simulink model "LAB5T2"  (R2018b)
settings: Solver=VariableStepAuto  StartTime=0.0  StopTime=100  RelTol=1e-3
settings Model: Creator=aloisia  LastModifiedBy=aloisia

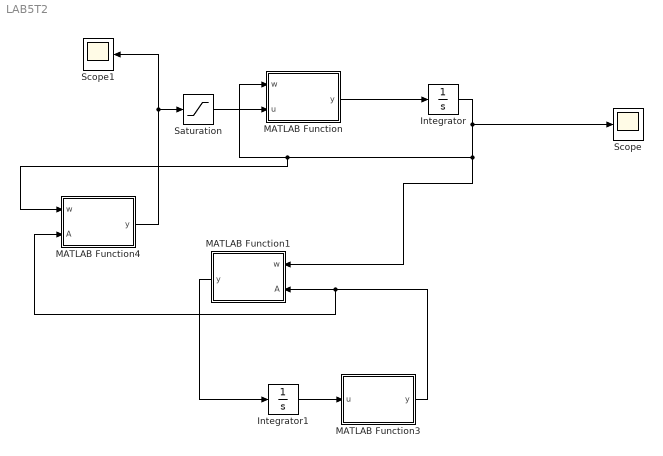
== system LAB5T2 ==
  Integrator : Integrator  InitialCondition=[0; 0; 0.01]
  Integrator1 : Integrator  InitialCondition=[-0.782 0 -0.6233;-0.6233 0 -0.782;0 -1 0]
  MATLAB Function : MATLAB Function  TreatAsAtomicUnit=on
  MATLAB Function1 : MATLAB Function  TreatAsAtomicUnit=on
  MATLAB Function3 : MATLAB Function  TreatAsAtomicUnit=on
  MATLAB Function4 : MATLAB Function  TreatAsAtomicUnit=on
  Saturation : Saturate  UpperLimit=0.01  LowerLimit=0.01
  Scope : Scope
  Scope1 : Scope
  wires:
  MATLAB Function3/1(y) -> MATLAB Function4/2(A), MATLAB Function1/2(A)
  MATLAB Function/1(y) -> Integrator/1
  Integrator1/1 -> MATLAB Function3/1(u)
  Integrator/1 -> MATLAB Function4/1(w), MATLAB Function/1(w), MATLAB Function1/1(w), Scope/1
  MATLAB Function1/1(y) -> Integrator1/1
  MATLAB Function4/1(y) -> Scope1/1, Saturation/1
  Saturation/1 -> MATLAB Function/2(u)

== matlab function LAB5T2/MATLAB Function1 ==
  data: w input; y output; A input
function y = Kinematic(w,A)

W=[0 -w(3) w(2);w(2) 0 -w(1);-w(2) w(1) 0];
Adot=-W*A;
y=Adot;
end

== matlab function LAB5T2/MATLAB Function ==
  data: w input; u input; y output
function y = Euler(w,u)
%First laboratory

%Datas
J1=0.01;
J2=0.05;
J3=0.07;

omx=w(1);
omy=w(2);
omz=w(3);

%Formula
omxdot=(J2-J3)/J1*omy*omz + u(1)/J1;
omydot=(J3-J1)/J2*omx*omz + u(2)/J2;
omzdot=(J1-J2)/J3*omy*omx + u(3)/J3;

y=[omxdot; omydot; omzdot];

end

== matlab function LAB5T2/MATLAB Function3 ==
  data: u input; y output
function y = Orthonorm(u)

t=abs(trace(eye(3)-u'*u));

    while t>0.00000001 
    A=(1.5)*u-u*u'*0.5*u;
    t=abs(trace(eye(3)-A'*A));
    u=A;
    end

y=u;
end

== matlab function LAB5T2/MATLAB Function4 ==
  data: w input; A input; y output
function y = control_law(w,A)

J1=0.01;
J2=0.05;
J3=0.07;

J = diag([J1,J2,J3]);

% Set k1 and k2 due to have a faster stabilization
k1 = 0.01;
k2 = 0.01;

K = k1 * J;
C = k2 * J;

% Set control matrix Ac
Ac = eye(3);
% Set error matrix Ae
Ae = A*(Ac');
d = (Ae'- Ae);
e = [d(3,2);d(1,3);d(2,1)];

u = - K*e - C*w;

y=u;
